simulink model "simplified_system_model"  (R2025a)
settings: Solver=VariableStepAuto  StartTime=0.0  StopTime=10.0  RelTol=1e-3
libraries: simulink x1
settings Model: Creator=techn  LastModifiedBy=techn

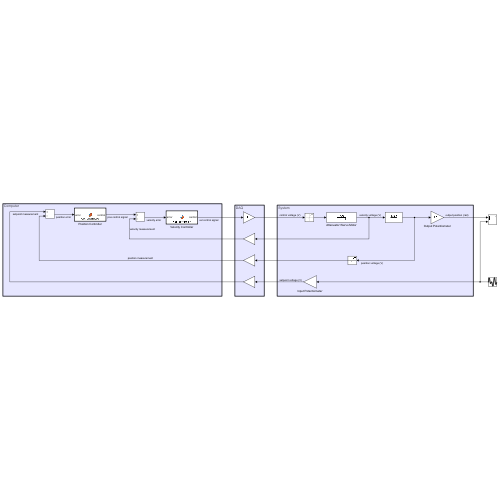
[thumbnail: Simulink's stored preview of the top-level diagram]
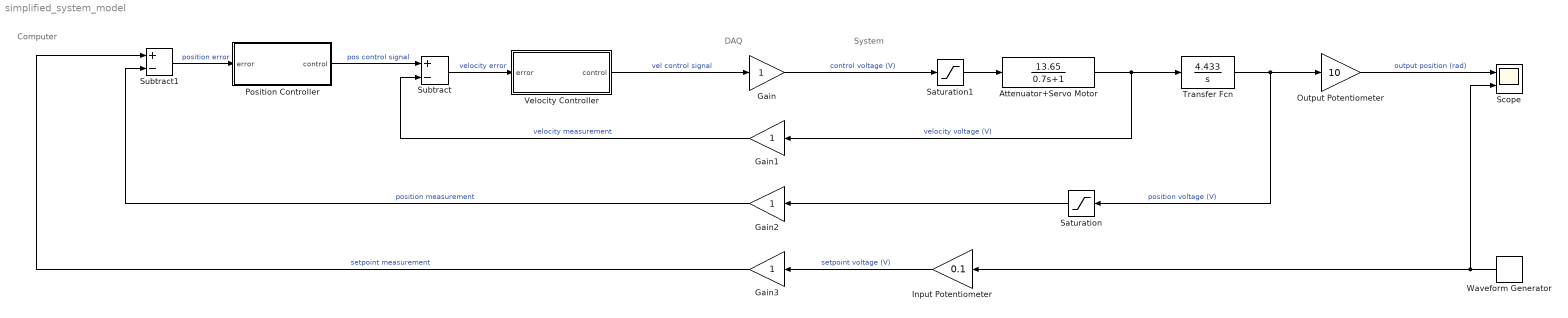
== system simplified_system_model ==
  note: System
  note: Computer
  note: DAQ
  Attenuator+Servo Motor : TransferFcn  Numerator=[13.65]  Denominator=[0.7,1]
  Gain{,1..3} (4 alike) : Gain
  Input Potentiometer : Gain  Gain=0.1
  Output Potentiometer : Gain  Gain=10
  Position Controller : MATLAB Function  TreatAsAtomicUnit=on
  Saturation : Saturate  UpperLimit=10  LowerLimit=-10
  Saturation1 : Saturate  UpperLimit=15  LowerLimit=-15
  Scope : Scope  NumInputPorts=2
  Subtract : Sum  Inputs=+-
  Subtract1 : Sum  Inputs=+-
  Transfer Fcn : TransferFcn  Numerator=[4.433]  Denominator=[1 0]
  Velocity Controller : MATLAB Function  TreatAsAtomicUnit=on
  Waveform Generator : simulink/Sources/Waveform Generator  OutMin=[]  OutMax=[]  OutDataTypeStr=double  SelectedSignal=1  BlockNames=MultiportSwitch_e3df3653d217406  SampleTime=0.1
  wires:
  Attenuator+Servo Motor/1 -> Gain1/1, Transfer Fcn/1  "velocity voltage (V)"
  Transfer Fcn/1 -> Saturation/1, Output Potentiometer/1  "position voltage (V)"
  Input Potentiometer/1 -> Gain3/1  "setpoint voltage (V)"
  Gain/1 -> Saturation1/1  "control voltage (V)"
  Velocity Controller/1(control) -> Gain/1  "vel control signal"
  Subtract/1 -> Velocity Controller/1(error)  "velocity error"
  Position Controller/1(control) -> Subtract/1  "pos control signal"
  Subtract1/1 -> Position Controller/1(error)  "position error"
  Gain3/1 -> Subtract1/1  "setpoint measurement"
  Gain1/1 -> Subtract/2  "velocity measurement"
  Gain2/1 -> Subtract1/2  "position measurement"
  Output Potentiometer/1 -> Scope/1  "output position (rad)"
  Waveform Generator/1 -> Input Potentiometer/1, Scope/2
  Saturation/1 -> Gain2/1
  Saturation1/1 -> Attenuator+Servo Motor/1

== matlab function simplified_system_model/Velocity Controller ==
  data: error input; control output
function control = vel_controller(error)
    control = error;
end

== matlab function simplified_system_model/Position Controller ==
  data: error input; control output
function control = pos_controller(error)
    control = error;
end
